simulink model "phdMain"  (R2023b)
settings: Solver=ode4  StartTime=0.0  StopTime=t.Data(end)  FixedStep=1e-3  RelTol=1e-3
values from neighbouring files (symbols this model uses):
  Am = T * Ac * inv(T)    [ref_model_mrac.m]
  Bm = T * Bc    [ref_model_mrac.m]
  Cm = eye(3)    [ref_model_mrac.m]
  Dm = zeros(3,1)    [ref_model_mrac.m]
undefined symbols (not defined in the file or in its folder): A_bar, AEFF, B_E, C_bar, C_T, Cd_neg, Cd_pos, DiscIntNeverNeededParam, Gamma, H, k, K, L_gain, L_STROKE, M, m3PsToLpm, P_return_Pa, P_supply_Pa, PA_Pa, PaToBar, PB_Pa, RHO, Ts, V01, V02, V_DEAD, v_mPs, W, xc_dot, xc_m
(part 1 of 3)
settings Model: PauseTimes=22  Creator=snr  LastModifiedBy=snr
settings DataIOCC: OutputOption=AdditionalOutputTimes  OutputTimes=1
settings OptimizationCC: BlockReduction=off  ConditionallyExecuteInputs=off
settings DebuggingCC: UnderSpecifiedDimensionMsg=warning

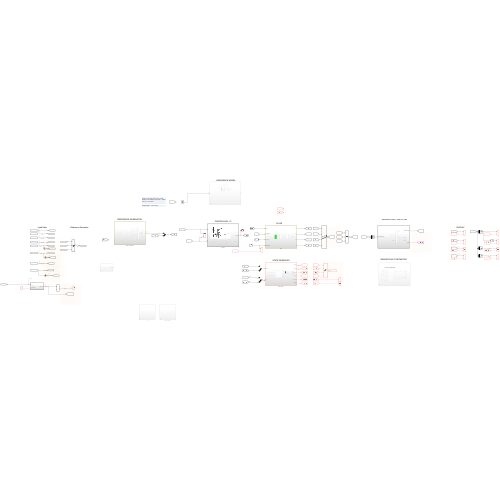
[thumbnail: Simulink's stored preview of the top-level diagram]
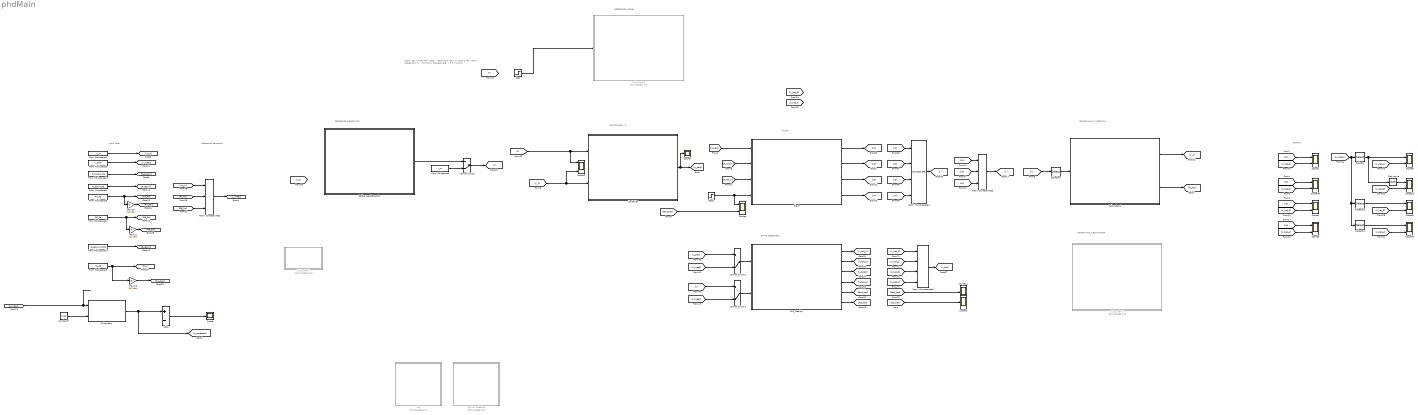
== system phdMain ==
  note: Kapalı Çevrim Faz Marjı (deg) > 6dB
      | Kapalı Çevrim Kazanç Marjı (dB) > 45deg
      | Aşım % < %5 olsun.
      |
      | Bantgenişliği > 5.5 Hz olsun
  note: Load Data
  note: PLANT
  note: CONTROLLER - PI
  note: DISPLAY
  note: Reference Generator
  note: SENSOR FAULT INJECTION
  note: STATE OBSERVER
  note: SENSOR FAULT ESTIMATOR
  note: REFERENCE GENERATOR
  note: REFERENCE MODEL
  Add5 : Sum  Inputs=+-
  Constant9 : Constant  Value=2.45
  Controller : Subsystem
  Derivative : Derivative
  EKF_Healthy : Subsystem
  From Workspace1 : FromWorkspace  VariableName=P_return_Pa
  From Workspace10 : FromWorkspace  VariableName=P_supply_Pa
  From Workspace11 : FromWorkspace  VariableName=PB_Pa
  From Workspace14 : FromWorkspace  VariableName=Q_return_m3Ps
  From Workspace2 : FromWorkspace  VariableName=r_m
  From Workspace3 : FromWorkspace  VariableName=u_perc
  From Workspace4 : FromWorkspace  VariableName=xc_m
  From Workspace5 : FromWorkspace  VariableName=PL_Pa
  From Workspace9 : FromWorkspace  VariableName=PA_Pa
  Gain19 : Gain  Gain=PaToBar
  Gain20 : Gain  Gain=PaToBar
  Gain21 : Gain  Gain=PaToBar
  Manual Switch : ManualSwitch  CurrentSetting=0
  Manual Switch1 : ManualSwitch  CurrentSetting=0
  Manual Switch2 : ManualSwitch  CurrentSetting=0
  Matrix Concatenate2 : Concatenate  NumInputs=3  Mode=Multidimensional array
  Matrix Concatenate3 : Concatenate  NumInputs=3  Mode=Multidimensional array
  Matrix Concatenate4 : Concatenate  NumInputs=4  Mode=Multidimensional array
  Matrix Concatenate5 : Concatenate  NumInputs=4  Mode=Multidimensional array
  Nguyen Observer : Subsystem  Commented=on
  Plant : Subsystem
  Reference_Generator : Subsystem
  Scope{,6..7,12} (4 alike) : Scope
  Scope{1..2,4..5,8..11,36} (9 alike) : Scope  NumInputPorts=2
  Scope3 : Scope  NumInputPorts=3
  Selector : Selector  InputPortWidth=3  IndexOptions=Index vector (dialog)  Indices=1  OutputSizes=1
  Selector1 : Selector  InputPortWidth=3  IndexOptions=Index vector (dialog)  Indices=3  OutputSizes=1
  Selector2 : Selector  InputPortWidth=3  IndexOptions=Index vector (dialog)  Indices=2  OutputSizes=1
  Selector4 : Selector  InputPortWidth=3  IndexOptions=Index vector (dialog)  Indices=1  OutputSizes=1
  Step : Step  After=10e-3  SampleTime=0
  Step2 : Step  Time=5  After=0  SampleTime=0
  Subsystem : Subsystem
  Subsystem1 : Subsystem
  Subsystem2 : Subsystem  Commented=on
  Subsystem3 : Subsystem  Commented=on
  Subsystem4 : Subsystem  Commented=on
  old : Subsystem  Commented=on
  wires:
  From Workspace3/1 -> [u_meas]  "u_real"
  From Workspace10/1 -> [P_supply]  "P_supply_Pa"
  From Workspace1/1 -> [P_return]  "P_return_Pa"
  From Workspace9/1 -> Gain20/1, [PA_Pa]  "PA_Pa"
  From Workspace11/1 -> Gain21/1, [PB_Pa]  "PB_Pa"
  From Workspace14/1 -> [Q_return]  "Q_return_m3Ps"
  From Workspace5/1 -> [P_L], Gain19/1  "P_L_Pa"
  Gain19/1 -> [P_L_bar]  "P_L_bar"
  Gain20/1 -> [PA_bar]  "PA_bar"
  Gain21/1 -> [PB_bar]  "PB_bar"
  [P_supply] -> Plant/2(P_supply_Pa)
  [P_return] -> Plant/3(P_return_Pa)
  Step2/1 -> Scope4/1, Plant/4(F_external_N)
  Plant/1(x1) -> [x1]
  Plant/2(x2) -> [x2]
  Plant/3(x3) -> [x3]
  Plant/4(x4) -> [x4]
  [x1] -> Matrix Concatenate3/1
  [x3] -> Matrix Concatenate3/2
  [x4] -> Matrix Concatenate3/3
  Matrix Concatenate3/1 -> [y]
  EKF_Healthy/1(x_hat_1) -> [x_hat_1]  "x_hat_1"
  EKF_Healthy/2(x_hat_2) -> [x_hat_2]  "x_hat_2"
  EKF_Healthy/3(x_hat_3) -> [x_hat_3]
  EKF_Healthy/4(x_hat_4) -> [x_hat_4]
  [x1] -> Matrix Concatenate4/1
  [x2] -> Matrix Concatenate4/2
  [x3] -> Matrix Concatenate4/3
  [x4] -> Matrix Concatenate4/4
  Matrix Concatenate4/1 -> [x]
  [x_hat_1] -> Matrix Concatenate5/1
  [x_hat_2] -> Matrix Concatenate5/2
  [x_hat_3] -> Matrix Concatenate5/3
  [x_hat_4] -> Matrix Concatenate5/4
  Matrix Concatenate5/1 -> [x_hat]
  EKF_Healthy/5(Fext_hat) -> [Fext_hat]
  EKF_Healthy/6(Qd_est) -> [Qd_hat]
  [x2] -> Scope36/1
  [x_hat_2] -> Scope36/2
  [y] -> Selector4/1
  Selector4/1 -> Subsystem1/1(Real_Cylinder_Pos)
  Subsystem1/1(Measured_Pos) -> [y_1]
  Subsystem1/2(fs_real) -> [fs_real]
  Controller/1(u_out_perc) -> Scope7/1, [u_perc]
  Step/1 -> Subsystem3/1(r)  "r"
  [y_1] -> Scope3/3, Controller/2(y)  "y_pid"
  Add5/1 -> Scope/1  "u_err"
  Subsystem/1(u_corrected) -> [u_corrected], Add5/1  "u_corrected"
  [u_meas] -> Subsystem/1(u)
  Constant9/1 -> Subsystem/2(u_perc_offset)
  [Fext_hat] -> Scope4/2
  Manual Switch/1 -> [r]  "r_m"
  Reference_Generator/1(r) -> Manual Switch/1  "r"
  From Workspace2/1 -> Manual Switch/2
  [x1] -> Scope1/1
  [x_hat_1] -> Scope1/2
  [x_hat_3] -> Scope2/2
  [x3] -> Scope2/1
  [x4] -> Scope5/1
  [x_hat_4] -> Scope5/2
  [Qd_hat] -> Scope6/1
  [PB_Pa] -> Matrix Concatenate2/3
  [PA_Pa] -> Matrix Concatenate2/2
  [xc_m] -> Matrix Concatenate2/1
  Matrix Concatenate2/1 -> [y_meas]
  Manual Switch1/1 -> EKF_Healthy/2(y_k)
  [y] -> Manual Switch1/1
  [y_meas] -> Manual Switch1/2
  Manual Switch2/1 -> EKF_Healthy/1(u_perc)
  [u_perc] -> Manual Switch2/1
  [u_meas] -> Manual Switch2/2
  [u_perc] -> Plant/1(u_perc)
  [r] -> Scope3/1, Controller/1(r)
  Selector1/1 -> Scope11/1  "P2_real"
  [x_hat_4] -> Scope11/2
  Selector/1 -> Derivative/1, Scope8/1
  [x_hat_1] -> Scope8/2
  [x_hat_2] -> Scope10/2
  Derivative/1 -> Scope10/1
  [x_hat_3] -> Scope9/2
  Selector2/1 -> Scope9/1  "P1_real"
  [y_meas] -> Selector1/1, Selector2/1, Selector/1
  From Workspace4/1 -> [xc_m]  "xc_m"
  [Fext_hat] -> Scope12/1

== system phdMain/Controller ==
  note: Kontrolcü kazançları Kp : 5 - Ki :40 test düzeneğinde, Sim ortamında uygunluk için böyle ayarladım
  note: Offset - Yapmaya İhtiyaç yok
  note: Integral Gain
  note: Proportional Gain
  r : Inport  OutDataTypeStr=double
  y : Inport  Port=2  OutDataTypeStr=double
  Add : Sum
  Add1 : Sum  Inputs=+-
  Add3 : Sum
  Constant : Constant  Value=10
  Constant1 : Constant  Value=5
  Constant2 : Constant  Value=0  OutDataTypeStr=double
  Gain1 : Gain  Gain=1000
  Integrator : Integrator
  Product : Product
  Product1 : Product
  Saturation : Saturate  UpperLimit=100  LowerLimit=-100
  u_out_perc : Outport  OutDataTypeStr=double
  wires:
  Constant/1 -> Product/1
  Constant1/1 -> Product1/1
  Add1/1 -> Product1/2, Product/2  "e"
  Product/1 -> Integrator/1
  Integrator/1 -> Add/2
  r/1 -> Add1/1  "r"
  Add/1 -> Gain1/1
  y/1 -> Add1/2
  Add3/1 -> Saturation/1
  Gain1/1 -> Add3/2
  Saturation/1 -> u_out_perc/1
  Product1/1 -> Add/1
  Constant2/1 -> Add3/1

== system phdMain/EKF_Healthy ==
  u_perc : Inport  OutDataTypeStr=double
  y_k : Inport  Port=2  OutDataTypeStr=double
  EKF_Discrete : MATLAB Function  TreatAsAtomicUnit=on  SystemSampleTime=1e-3
  Sel_d10 : Selector  InputPortWidth=6  IndexOptions=Index vector (dialog)  Indices=4  OutputSizes=1
  Sel_d7 : Selector  InputPortWidth=6  IndexOptions=Index vector (dialog)  Indices=1  OutputSizes=1
  Sel_d8 : Selector  InputPortWidth=6  IndexOptions=Index vector (dialog)  Indices=2  OutputSizes=1  RuntimeRangeChecks=on
  Sel_d9 : Selector  InputPortWidth=6  IndexOptions=Index vector (dialog)  Indices=3  OutputSizes=1
  Unit Delay : UnitDelay  SampleTime=1e-3  HasFrameUpgradeWarning=on
  x_hat_1 : Outport  OutDataTypeStr=double
  x_hat_2 : Outport  Port=2  OutDataTypeStr=double
  x_hat_3 : Outport  Port=3  OutDataTypeStr=double
  x_hat_4 : Outport  Port=4  OutDataTypeStr=double
  Fext_hat : Outport  Port=5  OutDataTypeStr=double
  Qd_est : Outport  Port=6  OutDataTypeStr=double
  wires:
  u_perc/1 -> EKF_Discrete/1(u_perc)  "u_perc"
  y_k/1 -> EKF_Discrete/2(y_k)
  EKF_Discrete/1(x_hat_out) -> Unit Delay/1
  Sel_d7/1 -> x_hat_1/1  "x_hat_1"
  Sel_d8/1 -> x_hat_2/1  "x_hat_2"
  Sel_d9/1 -> x_hat_3/1  "x_hat_3"
  Sel_d10/1 -> x_hat_4/1  "x_hat_4"
  EKF_Discrete/2(Fd_est) -> Fext_hat/1
  EKF_Discrete/3(Qd_est) -> Qd_est/1
  Unit Delay/1 -> Sel_d7/1, Sel_d10/1, Sel_d9/1, Sel_d8/1

== system phdMain/Nguyen Observer ==
  note: [1000; 1000; 1e-6; 1e-6]
  Add4 : Sum  Commented=on  Inputs=+-
  From Workspace13 : FromWorkspace  Commented=on  VariableName=P_return_Pa
  From Workspace16 : FromWorkspace  Commented=on  VariableName=P_supply_Pa
  From Workspace17 : FromWorkspace  Commented=on  VariableName=PB_Pa
  From Workspace18 : FromWorkspace  Commented=on  VariableName=PA_Pa
  From14 : From  Commented=on  GotoTag=u_perc
  From15 : From  Commented=on  GotoTag=xc_sim
  From20 : From  Commented=on  GotoTag=xc_dot_sim
  From29 : From  Commented=on  GotoTag=x1_hat
  From32 : From  Commented=on  GotoTag=xc_sim
  From33 : From  Commented=on  GotoTag=x2_hat
  From36 : From  Commented=on  GotoTag=fs_hat
  From37 : From  Commented=on  GotoTag=PA_sim_Pa
  From38 : From  Commented=on  GotoTag=x3_hat
  From40 : From  Commented=on  GotoTag=xc_dot_sim
  Gain15 : Gain  Commented=on  Gain=[1000; 1000; 1e-6; 1e-6]
  Goto21 : Goto  Commented=on  GotoTag=x1_hat
  Goto22 : Goto  Commented=on  GotoTag=x3_hat
  Goto26 : Goto  Commented=on  GotoTag=fs_hat
  Goto27 : Goto  Commented=on  GotoTag=x4_hat
  Goto28 : Goto  Commented=on  GotoTag=x2_hat
  Matrix Concatenate : Concatenate  Commented=on  NumInputs=4  Mode=Multidimensional array
  Nguyen_Observer : Subsystem  Commented=on
  Scope12 : Scope  Commented=on  NumInputPorts=2
  Scope17 : Scope  Commented=on  NumInputPorts=2
  Scope18 : Scope  Commented=on
  Scope19 : Scope  Commented=on
  Scope20 : Scope  Commented=on  NumInputPorts=2
  Selector : Selector  Commented=on  InputPortWidth=5  IndexOptions=Index vector (dialog)  Indices=1  OutputSizes=1
  Selector1 : Selector  Commented=on  InputPortWidth=5  IndexOptions=Index vector (dialog)  Indices=2  OutputSizes=1
  Selector2 : Selector  Commented=on  InputPortWidth=5  IndexOptions=Index vector (dialog)  Indices=3  OutputSizes=1
  Selector3 : Selector  Commented=on  InputPortWidth=5  IndexOptions=Index vector (dialog)  Indices=4  OutputSizes=1
  Selector4 : Selector  Commented=on  InputPortWidth=5  IndexOptions=Index vector (dialog)  Indices=5  OutputSizes=1
  Zero-Order Hold3 : ZeroOrderHold  Commented=on  SampleTime=Ts
  wires:
  From Workspace13/1 -> Nguyen_Observer/3(P_return)
  Add4/1 -> Scope19/1
  From Workspace17/1 -> Matrix Concatenate/4
  Selector4/1 -> Goto26/1
  From14/1 -> Nguyen_Observer/1(u_perc)  "u_perc"
  Selector2/1 -> Goto22/1
  Matrix Concatenate/1 -> Zero-Order Hold3/1
  From38/1 -> Scope20/2
  From Workspace16/1 -> Nguyen_Observer/2(P_supply)
  From32/1 -> Add4/1, Scope12/1
  Zero-Order Hold3/1 -> Gain15/1
  From36/1 -> Scope18/1
  From40/1 -> Scope17/1
  Gain15/1 -> Nguyen_Observer/4(y)
  From20/1 -> Matrix Concatenate/2
  From15/1 -> Matrix Concatenate/1
  Selector/1 -> Goto21/1
  Selector3/1 -> Goto27/1
  From37/1 -> Scope20/1  "PA_sim_Pa"
  Selector1/1 -> Goto28/1
  From Workspace18/1 -> Matrix Concatenate/3
  Nguyen_Observer/1(xbar_hat_safe) -> Selector4/1, Selector3/1, Selector2/1, Selector1/1, Selector/1
  From33/1 -> Scope17/2
  From29/1 -> Add4/2, Scope12/2

== system phdMain/Plant ==
  u_perc : Inport  OutDataTypeStr=double
  P_supply_Pa : Inport  Port=2
  P_return_Pa : Inport  Port=3
  F_external_N : Inport  Port=4
  Cylinder_Dynamics : Subsystem
  Pressure_Dynamics : Subsystem
  Subsystem1 : Subsystem
  x1 : Outport
  x2 : Outport  Port=2
  x3 : Outport  Port=3
  x4 : Outport  Port=4
  wires:
  Cylinder_Dynamics/1(xc_sim) -> [xc_sim]  "xc_sim_m"
  [xc_sim] -> Pressure_Dynamics/3(xc)
  P_supply_Pa/1 -> Subsystem1/2(P_supply)
  [PA_sim_Pa] -> Subsystem1/4(PA_sim_Pa)  "PA_sim_Pa"
  [PB_sim_Pa] -> Subsystem1/5(PB_sim_Pa)  "PB_sim_Pa"
  [PB_sim_Pa] -> Cylinder_Dynamics/2(PB_sim_Pa)  "PB_sim_Pa"
  Pressure_Dynamics/1(PA_sim) -> [PA_sim_Pa]  "PA_sim_Pa"
  Cylinder_Dynamics/3(xc_ddot_sim) -> [xc_ddot_sim]  "xc_ddot_sim_mPs2"
  Cylinder_Dynamics/2(xc_dot_sim) -> [xc_dot_sim]  "xc_dot_sim_mPs"
  [xc_dot_sim] -> Pressure_Dynamics/2(xc_dot)
  [PA_sim_Pa] -> Cylinder_Dynamics/1(PA_sim_Pa)  "PA_sim_Pa"
  Pressure_Dynamics/2(PB_sim) -> [PB_sim_Pa]  "PB_sim_Pa"
  Subsystem1/1(q_withLeaks) -> [Q_Bus]
  [Q_Bus] -> Pressure_Dynamics/1(q)
  u_perc/1 -> Subsystem1/1(u_perc)  "u_perc"
  P_return_Pa/1 -> Subsystem1/3(P_return)
  F_external_N/1 -> Cylinder_Dynamics/3(F_ext)
  [xc_sim] -> x1/1  "xc_sim"
  [xc_dot_sim] -> x2/1  "xc_dot_sim"
  [PA_sim_Pa] -> x3/1  "PA_sim_Pa"
  [PB_sim_Pa] -> x4/1  "PB_sim_Pa"

== system phdMain/Reference_Generator ==
  Constant : Constant  OutDataTypeStr=uint8
  Constant1 : Constant  Commented=on  Value=30  OutDataTypeStr=double
  Constant2 : Constant  Commented=on  OutDataTypeStr=double
  Constant3 : Constant  Commented=on  Value=0  OutDataTypeStr=double
  Constant4 : Constant  Value=0
  From Workspace14 : FromWorkspace  VariableName=r_m
  Gain : Gain
  Multiport Switch : MultiPortSwitch  DataPortOrder=Zero-based contiguous  DataPortForDefault=Additional data port  DiagnosticForDefault=None  zeroidx=on  OutDataTypeStr=double  SaturateOnIntegerOverflow=off  InputSameDT=off
  Pulse Generator : DiscretePulseGenerator  PulseType=Time based  Amplitude=20e-3  Period=4  PulseWidth=25
  Scope : Scope
  Sine Wave : Sin  Amplitude=30e-3  Frequency=pi*0.5  SampleTime=0
  Sine_Generator : Subsystem  Commented=on
  r : Outport  OutDataTypeStr=double
  wires:
  From Workspace14/1 -> Multiport Switch/2  "r_m"
  Constant/1 -> Multiport Switch/1
  Constant1/1 -> Sine_Generator/1(Amp_mm)
  Constant2/1 -> Sine_Generator/2(f_Hz)
  Constant3/1 -> Sine_Generator/3(phi_deg)
  Pulse Generator/1 -> Gain/1
  Multiport Switch/1 -> Scope/1, r/1
  Constant4/1 -> Multiport Switch/5
  Sine Wave/1 -> Multiport Switch/3
  Gain/1 -> Multiport Switch/4

== system phdMain/Subsystem ==
  u : Inport  OutDataTypeStr=double
  u_perc_offset : Inport  Port=2  OutDataTypeStr=double
  Add : Sum  Inputs=+-
  u_corrected : Outport
  wires:
  u/1 -> Add/1
  u_perc_offset/1 -> Add/2
  Add/1 -> u_corrected/1

== system phdMain/Subsystem1 ==
  Real_Cylinder_Pos : Inport  OutDataTypeStr=double
  Add4 : Sum
  Fault_Injection : Subsystem  Commented=on
  Measured_Pos : Outport  OutDataTypeStr=double
  fs_real : Outport  Port=2  OutDataTypeStr=double
  wires:
  Fault_Injection/1(fs) -> [fs_real], Add4/1
  Real_Cylinder_Pos/1 -> Add4/2
  Add4/1 -> Measured_Pos/1  "y_1"
  [fs_real] -> fs_real/1

== system phdMain/Subsystem2 ==
  note: FAULT ESTIMATOR
  From14 : From  Commented=on  GotoTag=u_perc
  From15 : From  Commented=on  GotoTag=PA_sim_Pa
  From20 : From  Commented=on  GotoTag=PB_sim_Pa
  From29 : From  Commented=on  GotoTag=fs_real
  From33 : From  Commented=on  GotoTag=xc_dot_sim
  Scope12 : Scope  Commented=on  NumInputPorts=3
  Scope17 : Scope  Commented=on  NumInputPorts=3
  Subsystem3 : Subsystem  Commented=on
  wires:
  Subsystem3/2(Out1) -> Scope17/1
  From20/1 -> Subsystem3/3(PB_Pa)  "PB_sim_Pa"
  From29/1 -> Subsystem3/5(fs_real)
  From14/1 -> Subsystem3/1(u_real)  "u_perc"
  From33/1 -> Scope17/2
  From15/1 -> Subsystem3/2(PA_Pa)
  Subsystem3/1(x_bar) -> Scope12/2  "x_bar"

== system phdMain/Subsystem3 ==
  r : Inport  OutDataTypeStr=double
  Add : Sum  Inputs=+-
  Gain : Gain
  Scope10 : Scope  NumInputPorts=2
  Scope11 : Scope
  Scope12 : Scope
  Scope13 : Scope
  Scope8 : Scope  NumInputPorts=2
  Scope9 : Scope  NumInputPorts=2
  Selector : Selector  InputPortWidth=3  IndexOptions=Index vector (dialog)  Indices=1  OutputSizes=1
  Selector1 : Selector  InputPortWidth=3  IndexOptions=Index vector (dialog)  Indices=2  OutputSizes=1
  Selector2 : Selector  InputPortWidth=3  IndexOptions=Index vector (dialog)  Indices=3  OutputSizes=1
  State-Space : StateSpace  A=Am  B=Bm  C=Cm  D=Dm  InitialCondition=[0;0;0]
  Out1 : Outport
  wires:
  r/1 -> State-Space/1, Scope12/1, Scope8/1  "r"
  Selector1/1 -> Scope13/1, Scope9/1
  [x2] -> Scope9/2
  Gain/1 -> Scope10/1
  State-Space/1 -> Selector2/1, Selector1/1, Selector/1
  Selector/1 -> Scope8/2  "y_m"
  Selector2/1 -> Scope11/1, Gain/1
  Add/1 -> Scope10/2

== system phdMain/Subsystem4 ==
  In1 : Inport
  Add : Sum
  Constant : Constant
  Constant1 : Constant  Value=100
  Relational Operator : RelationalOperator  OutDataTypeStr=boolean  RndMeth=Simplest  InputSameDT=off
  Saturation : Saturate  UpperLimit=100  LowerLimit=0
  Switch : Switch  Criteria=u2 ~= 0  SaturateOnIntegerOverflow=off  InputSameDT=off
  Unit Delay : UnitDelay  SampleTime=-1  HasFrameUpgradeWarning=on
  u_perc_offset : Outport
  wires:
  Constant/1 -> Add/1
  Add/1 -> Unit Delay/1, Saturation/1
  Unit Delay/1 -> Add/2
  Saturation/1 -> Relational Operator/1
  Constant1/1 -> Relational Operator/2
  Relational Operator/1 -> Switch/2
  In1/1 -> Switch/1

== system phdMain/old ==
  Bus Creator1 : BusCreator  Commented=on  Inputs=3
  Constant10 : Constant  Commented=on  Value=mean(P_supply_Pa)
  Constant4 : Constant  Commented=on  Value=mean(P_return_Pa)
  Constant6 : Constant  Commented=on  Value=mean(P_supply_Pa)
  Constant9 : Constant  Commented=on  Value=mean(P_return_Pa)
  Flow_Calc_NoLeak : Subsystem  Commented=on
  Flow_Calc_WithLeak : Subsystem  Commented=on
  From Workspace13 : FromWorkspace  Commented=on  VariableName=P_supply_Pa
  From Workspace8 : FromWorkspace  Commented=on  VariableName=P_return_Pa
  From13 : From  Commented=on  GotoTag=PA_sim_Pa
  From14 : From  Commented=on  GotoTag=PB_sim_Pa
  From15 : From  Commented=on  GotoTag=u_perc
  From23 : From  Commented=on  GotoTag=PA_sim_Pa
  From26 : From  Commented=on  GotoTag=PB_sim_Pa
  From29 : From  Commented=on  GotoTag=Q_return
  From32 : From  Commented=on  GotoTag=q_withLeaks
  From37 : From  Commented=on  GotoTag=xv
  From38 : From  Commented=on  GotoTag=PA_sim_Pa
  From39 : From  Commented=on  GotoTag=PB_sim_Pa
  From40 : From  Commented=on  GotoTag=xv
  From43 : From  Commented=on  GotoTag=xv
  Gain15 : Gain  Commented=on  Gain=50E-3/100
  Gain16 : Gain  Commented=on  Gain=m3PsToLpm
  Gain17 : Gain  Commented=on  Gain=m3PsToLpm
  Goto21 : Goto  Commented=on  GotoTag=xv
  Goto26 : Goto  Commented=on  GotoTag=q_withLeaks
  Goto27 : Goto  Commented=on  GotoTag=q_NoLeaks
  MATLAB Function2 : MATLAB Function  Commented=on  TreatAsAtomicUnit=on
  Scope14 : Scope  NumInputPorts=2
  Scope17 : Scope  Commented=on  NumInputPorts=2
  ServoValve_Dynamics : Subsystem  Commented=on
  wires:
  Constant9/1 -> MATLAB Function2/3(P_T)
  From32/1 -> Scope14/2
  Constant4/1 -> Flow_Calc_WithLeak/3(P_return)
  From26/1 -> MATLAB Function2/5(P_B)  "PB_sim_Pa"
  From Workspace13/1 -> Flow_Calc_NoLeak/2(P_supply)
  From29/1 -> Gain17/1
  Gain15/1 -> MATLAB Function2/1(xv)
  Bus Creator1/1 -> Scope14/1
  From37/1 -> Flow_Calc_WithLeak/1(xv)
  Constant10/1 -> MATLAB Function2/2(P_P)
  From Workspace8/1 -> Flow_Calc_NoLeak/3(P_return)
  MATLAB Function2/3(Q_RETURN) -> Gain16/1, Bus Creator1/3  "Q_RETURN_lpm"
  From23/1 -> MATLAB Function2/4(P_A)  "PA_sim_Pa"
  Gain16/1 -> Scope17/2  "Q_RETURN_lpm"
  MATLAB Function2/1(Q1) -> Bus Creator1/1  "q1"
  MATLAB Function2/2(Q2) -> Bus Creator1/2  "q2"
  From14/1 -> Flow_Calc_WithLeak/5(P_2)  "P_2_sim"
  From39/1 -> Flow_Calc_NoLeak/5(P_2)  "P_2_sim"
  Flow_Calc_NoLeak/1(Q) -> Goto27/1
  Flow_Calc_WithLeak/1(q_withLeaks) -> Goto26/1
  From40/1 -> Flow_Calc_NoLeak/1(xv)
  [u_sim] -> Gain15/1
  Constant6/1 -> Flow_Calc_WithLeak/2(P_supply)
  From38/1 -> Flow_Calc_NoLeak/4(P_1)  "P_1_sim"
  From13/1 -> Flow_Calc_WithLeak/4(P_1)  "P_1_sim"
  Gain17/1 -> Scope17/1  "Q_RETURN_lpmREAL"
  ServoValve_Dynamics/1(xv) -> Goto21/1  "xv"
  From15/1 -> ServoValve_Dynamics/1(u)  "u_sim"

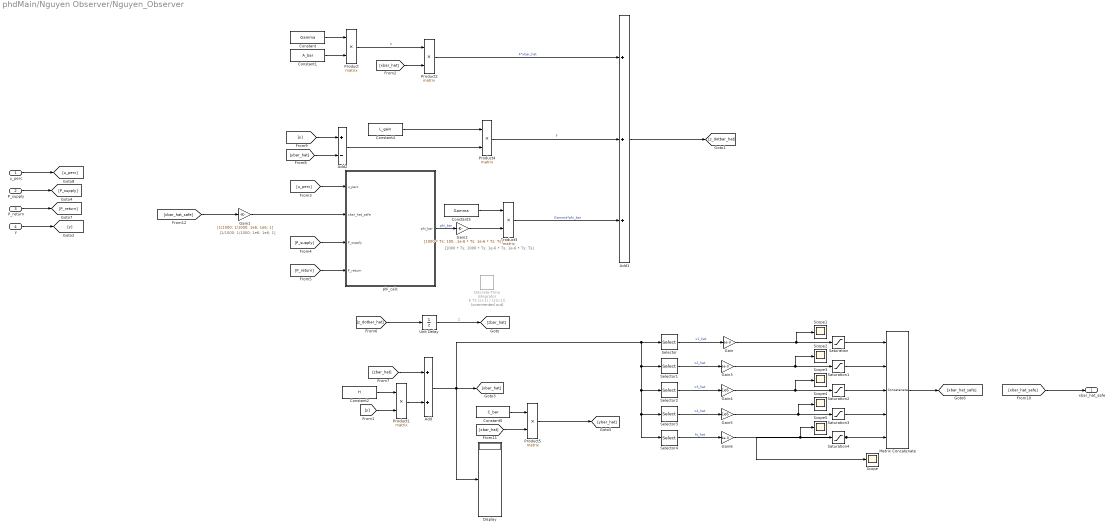
== system phdMain/Nguyen Observer/Nguyen_Observer ==
  note: [1000 * Ts; 1000 * Ts; 1e-6 * Ts; 1e-6 * Ts; Ts]
  note: [1/1000; 1/1000; 1e6; 1e6; 1]
  u_perc : Inport  PortDimensions=[1,1]
  P_supply : Inport  Port=2  OutDataTypeStr=double
  P_return : Inport  Port=3  OutDataTypeStr=double
  y : Inport  Port=4  PortDimensions=[4,1]
  Add : Sum
  Add1 : Sum  Inputs=+++
  Add2 : Sum  Inputs=+-
  Constant : Constant  Value=Gamma
  Constant1 : Constant  Value=A_bar
  Constant2 : Constant  Value=H
  Constant3 : Constant  Value=Gamma
  Constant4 : Constant  Value=L_gain
  Constant5 : Constant  Value=C_bar
  Discrete-Time Integrator : DiscreteIntegrator  Commented=on  IntegratorMethod=Integration: Trapezoidal  InitialCondition=[0,0,PA_Pa.Data(1)*1e-6,PB_Pa.Data(1)*1e-6,0]'  SampleTime=-1  ICPrevOutput=DiscIntNeverNeededParam  ICPrevScaledInput=DiscIntNeverNeededParam
  Display : Display
  Gain : Gain  Gain=1e-3
  Gain1 : Gain  Gain=[1/1000; 1/1000; 1e6; 1e6; 1]
  Gain2 : Gain  Gain=[1000 * Ts; 1000 * Ts; 1e-6 * Ts; 1e-6 * Ts; Ts]
  Gain3 : Gain  Gain=1e-3
  Gain4 : Gain  Gain=1e6
  Gain5 : Gain  Gain=1e6
  Gain6 : Gain  Gain=1e-3
  Matrix Concatenate : Concatenate  NumInputs=5  Mode=Multidimensional array
  Product{,1..5} (6 alike) : Product  Multiplication=Matrix(*)
  Saturation : Saturate  UpperLimit=L_STROKE  LowerLimit=-L_STROKE
  Saturation1 : Saturate  UpperLimit=2  LowerLimit=-2
  Saturation2 : Saturate  UpperLimit=200e5  LowerLimit=4e5
  Saturation3 : Saturate  UpperLimit=200e5  LowerLimit=4e5
  Saturation4 : Saturate  UpperLimit=L_STROKE  LowerLimit=-L_STROKE
  Scope{,1..5} (6 alike) : Scope
  Selector : Selector  InputPortWidth=5  IndexOptions=Index vector (dialog)  Indices=1  OutputSizes=1
  Selector1 : Selector  InputPortWidth=5  IndexOptions=Index vector (dialog)  Indices=2  OutputSizes=1
  Selector2 : Selector  InputPortWidth=5  IndexOptions=Index vector (dialog)  Indices=3  OutputSizes=1
  Selector3 : Selector  InputPortWidth=5  IndexOptions=Index vector (dialog)  Indices=4  OutputSizes=1
  Selector4 : Selector  InputPortWidth=5  IndexOptions=Index vector (dialog)  Indices=5  OutputSizes=1
  Unit Delay : UnitDelay  InitialCondition=[0,0,PA_Pa.Data(1)*1e-6,PB_Pa.Data(1)*1e-6,0]'  SampleTime=Ts  HasFrameUpgradeWarning=on
  phi_calc : Subsystem
  xbar_hat_safe : Outport
  wires:
  [y] -> Add2/1
  Product3/1 -> Add1/3  "Gamma*phi_bar"
  [u_perc] -> phi_calc/1(u_perc)
  Add2/1 -> Product4/2
  u_perc/1 -> [u_perc]
  Constant3/1 -> Product3/1
  Unit Delay/1 -> [zbar_hat]  "z"
  [ybar_hat] -> Add2/2
  Constant2/1 -> Product1/1
  Product/1 -> Product2/1  "F"
  [P_return] -> phi_calc/4(P_return)
  Constant1/1 -> Product/2
  Product2/1 -> Add1/1  "F*xbar_hat"
  Constant/1 -> Product/1
  [xbar_hat] -> Product2/2
  P_return/1 -> [P_return]
  [y] -> Product1/2
  [zbar_hat] -> Add/1
  y/1 -> [y]
  Add1/1 -> [z_dotbar_hat]
  Product4/1 -> Add1/2  "F"
  Product1/1 -> Add/2
  P_supply/1 -> [P_supply]
  phi_calc/1(phi_bar) -> Gain2/1  "phi_bar"
  [P_supply] -> phi_calc/3(P_supply)
  [z_dotbar_hat] -> Unit Delay/1
  [xbar_hat_safe] -> xbar_hat_safe/1
  Constant5/1 -> Product5/1
  [xbar_hat] -> Product5/2
  Product5/1 -> [ybar_hat]
  Selector3/1 -> Gain5/1  "x4_hat"
  Selector2/1 -> Gain4/1  "x3_hat"
  Selector1/1 -> Gain3/1  "x2_hat"
  Saturation/1 -> Matrix Concatenate/1
  Saturation1/1 -> Matrix Concatenate/2
  Saturation2/1 -> Matrix Concatenate/3
  Saturation3/1 -> Matrix Concatenate/4
  Saturation4/1 -> Scope/1, Matrix Concatenate/5
  Matrix Concatenate/1 -> [xbar_hat_safe]
  Selector4/1 -> Gain6/1  "fs_hat"
  Selector/1 -> Gain/1  "x1_hat"
  Constant4/1 -> Product4/1
  Add/1 -> Selector3/1, Selector4/1, Selector2/1, Selector1/1, Selector/1, [xbar_hat], Display/1
  [xbar_hat_safe] -> Gain1/1
  Gain1/1 -> phi_calc/2(xbar_hat_safe)
  Gain2/1 -> Product3/2
  Gain/1 -> Scope1/1, Saturation/1
  Gain3/1 -> Scope2/1, Saturation1/1
  Gain4/1 -> Saturation2/1, Scope3/1
  Gain5/1 -> Saturation3/1, Scope4/1
  Gain6/1 -> Scope5/1, Saturation4/1

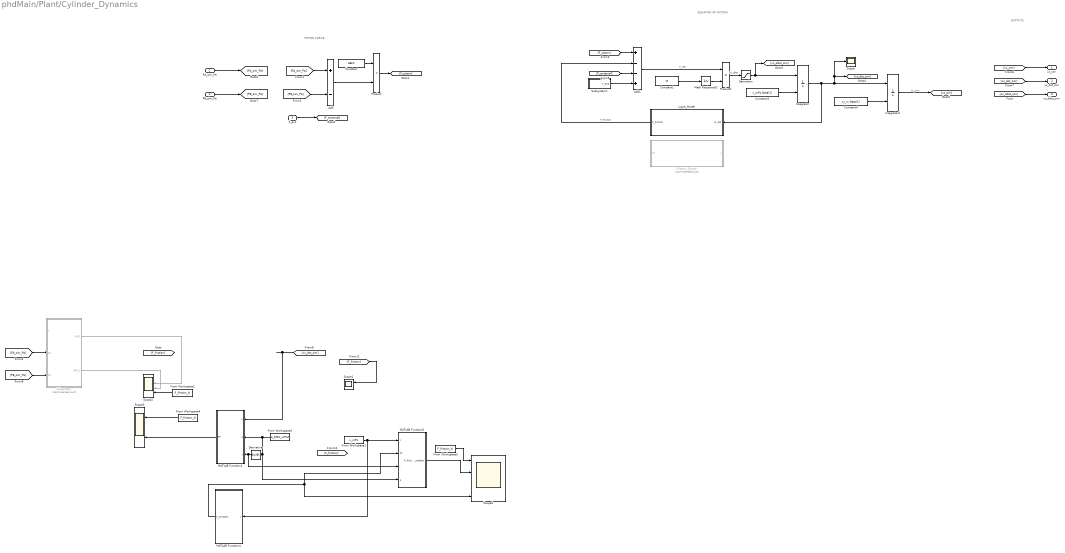
== system phdMain/Plant/Cylinder_Dynamics ==
  note: PISTON FORCE
  note: EQUATION OF MOTION
  note: OUTPUTS
  PA_sim_Pa : Inport  OutDataTypeStr=double
  PB_sim_Pa : Inport  Port=2  OutDataTypeStr=double
  F_ext : Inport  Port=3  OutDataTypeStr=double
  Add : Sum  Inputs=+-
  Add1 : Sum  Inputs=+--+
  Constant : Constant  Value=AEFF  OutDataTypeStr=double
  Constant1 : Constant  Value=M  OutDataTypeStr=double
  Constant3 : Constant  Value=v_mPs.Data(1)
  Constant4 : Constant  Value=xc_m.Data(1)
  Derivative : Derivative
  Friction_Simple : MATLAB Function  Commented=on  TreatAsAtomicUnit=on
  From Workspace1 : FromWorkspace  VariableName=v_mPs
  From Workspace2 : FromWorkspace  VariableName=F_friction_N
  From Workspace3 : FromWorkspace  VariableName=F_friction_N
  From Workspace4 : FromWorkspace  VariableName=F_friction_N
  From Workspace5 : FromWorkspace  VariableName=a_RMC_mPs2
  Integrator : Integrator  InitialConditionSource=external  InitialCondition=xc_dot(1)  UpperSaturationLimit=4  LowerSaturationLimit=-4
  Integrator2 : Integrator  InitialConditionSource=external  InitialCondition=xc_dot(1)  LimitOutput=on  UpperSaturationLimit=0.09580  LowerSaturationLimit=-0.09580
  Lugre_Model : Subsystem
  MATLAB Function1 : MATLAB Function  TreatAsAtomicUnit=on
  MATLAB Function3 : MATLAB Function  TreatAsAtomicUnit=on
  MATLAB Function4 : MATLAB Function  TreatAsAtomicUnit=on
  Math Reciprocal2 : Math  Operator=reciprocal  SignedPower=on
  Product : Product
  Product1 : Product
  Saturation : Saturate  UpperLimit=100  LowerLimit=-100
  Scope : Scope
  Scope1 : Scope  NumInputPorts=2
  Scope2 : Scope  NumInputPorts=6
  Scope3 : Scope  NumInputPorts=2
  Scope4 : Scope  NumInputPorts=4
  Subsystem : Subsystem  Commented=on
  Subsystem1 : Subsystem
  xc_sim : Outport  OutDataTypeStr=double
  xc_dot_sim : Outport  Port=2  OutDataTypeStr=double
  xc_ddot_sim : Outport  Port=3  OutDataTypeStr=double
  wires:
  [PB_sim_Pa] -> Add/2
  [PA_sim_Pa] -> Add/1
  Add/1 -> Product/2
  Constant/1 -> Product/1
  Math Reciprocal2/1 -> Product1/2
  Product1/1 -> Saturation/1  "xc_ddot"
  Product/1 -> [F_piston]
  F_ext/1 -> [F_external]
  Add1/1 -> Product1/1  "F_net"
  Constant3/1 -> Integrator/2
  Integrator/1 -> Integrator2/1, Scope/1, [xc_dot_sim], Lugre_Model/1(xc_dot)
  Constant4/1 -> Integrator2/2
  Integrator2/1 -> [xc_sim]  "xc_sim"
  [xc_sim] -> xc_sim/1
  [xc_dot_sim] -> xc_dot_sim/1
  [xc_dot_sim] -> MATLAB Function1/1(v)
  [xc_ddot_sim] -> xc_ddot_sim/1
  Saturation/1 -> [xc_ddot_sim], Integrator/1
  [F_external] -> Add1/3
  [F_piston] -> Add1/1
  ? -> Scope2/1, [F_friction]  "F_friction"
  From Workspace2/1 -> Scope2/5
  Subsystem1/1(F_end) -> Add1/4
  PA_sim_Pa/1 -> [PA_sim_Pa]
  PB_sim_Pa/1 -> [PB_sim_Pa]
  [PA_sim_Pa] -> Subsystem/2(pa)
  [PB_sim_Pa] -> Subsystem/3(pb)
  Constant1/1 -> Math Reciprocal2/1
  Subsystem/2(FRIC1) -> Scope2/4
  Subsystem/1(FRIC) -> Scope2/3
  Derivative/1 -> MATLAB Function3/3(j), MATLAB Function1/3(j)
  From Workspace4/1 -> Scope3/1
  MATLAB Function1/1(FF) -> Scope3/2
  From Workspace5/1 -> MATLAB Function3/4(a), Derivative/1, MATLAB Function1/2(a)
  [F_friction] -> Scope1/1
  From Workspace1/1 -> MATLAB Function4/1(v), MATLAB Function3/1(v)
  MATLAB Function3/1(F_friction_nodelay) -> Scope4/2
  From Workspace3/1 -> Scope4/1
  MATLAB Function4/1(F_stribeck) -> MATLAB Function3/2(FF), Scope4/4
  Lugre_Model/1(F_friction) -> Add1/2  "F_friction"

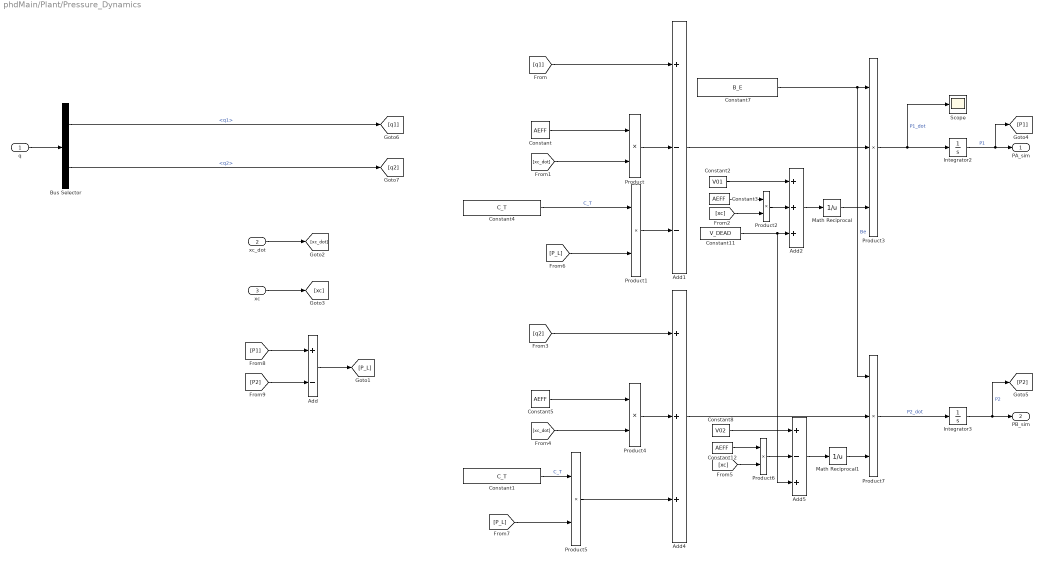
== system phdMain/Plant/Pressure_Dynamics ==
  q : Inport  OutDataTypeStr=double
  xc_dot : Inport  Port=2  OutDataTypeStr=double
  xc : Inport  Port=3  OutDataTypeStr=double
  Add : Sum  Inputs=+-
  Add1 : Sum  Inputs=+--
  Add2 : Sum  Inputs=+++
  Add4 : Sum  Inputs=+++
  Add5 : Sum  Inputs=+-+
  Bus Selector : BusSelector  OutputSignals=q1,q2
  Constant{,3,5,12} (4 alike) : Constant  Value=AEFF  OutDataTypeStr=double
  Constant1 : Constant  Value=C_T  OutDataTypeStr=double
  Constant11 : Constant  Value=V_DEAD  OutDataTypeStr=double
  Constant2 : Constant  Value=V01  OutDataTypeStr=double
  Constant4 : Constant  Value=C_T  OutDataTypeStr=double
  Constant7 : Constant  Value=B_E  OutDataTypeStr=double
  Constant8 : Constant  Value=V02  OutDataTypeStr=double
  Integrator2 : Integrator  InitialCondition=PA_Pa.Data(1)  LimitOutput=on  UpperSaturationLimit=200e5  LowerSaturationLimit=4e5
  Integrator3 : Integrator  InitialCondition=PB_Pa.Data(1)  LimitOutput=on  UpperSaturationLimit=200e5  LowerSaturationLimit=4e5
  Math Reciprocal : Math  Operator=reciprocal  SignedPower=on
  Math Reciprocal1 : Math  Operator=reciprocal  SignedPower=on
  Product{,1..2,4..6} (6 alike) : Product
  Product3 : Product  Inputs=3
  Product7 : Product  Inputs=3
  Scope : Scope
  PA_sim : Outport  OutDataTypeStr=double
  PB_sim : Outport  Port=2  OutDataTypeStr=double
  wires:
  q/1 -> Bus Selector/1
  xc_dot/1 -> [xc_dot]
  [xc_dot] -> Product/2
  Constant/1 -> Product/1
  Integrator2/1 -> [P1], PA_sim/1  "P1"
  [P_L] -> Product1/2
  Product/1 -> Add1/2
  [q1] -> Add1/1
  xc/1 -> [xc]
  Constant2/1 -> Add2/1
  Product2/1 -> Add2/2
  [xc] -> Product2/2
  Constant3/1 -> Product2/1
  Add2/1 -> Math Reciprocal/1
  Product3/1 -> Integrator2/1, Scope/1  "P1_dot"
  Math Reciprocal/1 -> Product3/3
  Add1/1 -> Product3/2
  Constant7/1 -> Product7/1, Product3/1  "Be"
  Constant4/1 -> Product1/1  "C_T"
  [xc_dot] -> Product4/2
  Product4/1 -> Add4/2
  Add4/1 -> Product7/2
  Integrator3/1 -> [P2], PB_sim/1  "P2"
  [P_L] -> Product5/2
  Constant5/1 -> Product4/1
  Add5/1 -> Math Reciprocal1/1
  [q2] -> Add4/1
  Math Reciprocal1/1 -> Product7/3
  Product7/1 -> Integrator3/1  "P2_dot"
  [xc] -> Product6/2
  Constant8/1 -> Add5/1
  Constant12/1 -> Product6/1
  Product6/1 -> Add5/2
  Bus Selector/2 -> [q2]  "<q2>"
  Bus Selector/1 -> [q1]  "<q1>"
  [P2] -> Add/2
  [P1] -> Add/1
  Add/1 -> [P_L]
  Constant1/1 -> Product5/1  "C_T"
  Product5/1 -> Add4/3
  Product1/1 -> Add1/3
  Constant11/1 -> Add5/3, Add2/3

== system phdMain/Plant/Subsystem1 ==
  u_perc : Inport  OutDataTypeStr=double
  P_supply : Inport  Port=2  OutDataTypeStr=double
  P_return : Inport  Port=3  OutDataTypeStr=double
  PA_sim_Pa : Inport  Port=4  OutDataTypeStr=double
  PB_sim_Pa : Inport  Port=5  OutDataTypeStr=double
  Bus Creator4 : BusCreator  Inputs=2
  Constant1 : Constant  Value=0.01
  Constant2 : Constant  Value=25e-3
  Constant4 : Constant  Value=k
  Constant7 : Constant  Value=K
  Dead Zone : DeadZone  LowerValue=-0.02  UpperValue=0.02
  Dead Zone1 : DeadZone  LowerValue=-0.02  UpperValue=0.02
  From Workspace2 : FromWorkspace  VariableName=Q_return_m3Ps
  Gain1 : Gain  Gain=m3PsToLpm
  Gain2 : Gain  Gain=m3PsToLpm
  MATLAB Function : MATLAB Function  TreatAsAtomicUnit=on
  Product : Product  Inputs=3
  Scope1 : Scope  NumInputPorts=2
  Terminator : Terminator
  Valve Dynamics : TransferFcn  Numerator=[2.0884e+06]  Denominator=[1 2*1*1.4451e+03 2.0884e+06]
  q_withLeaks : Outport  OutDataTypeStr=double
  wires:
  PA_sim_Pa/1 -> [P_A]
  P_supply/1 -> [P_supply]
  P_return/1 -> [P_return]
  PB_sim_Pa/1 -> [P_B]
  u_perc/1 -> [u_perc]
  [P_supply] -> MATLAB Function/2(Ps)
  [P_return] -> MATLAB Function/3(Pr)
  [P_A] -> MATLAB Function/4(P1)
  [P_B] -> MATLAB Function/5(P2)
  Bus Creator4/1 -> q_withLeaks/1
  MATLAB Function/1(Q1) -> Bus Creator4/1  "q1"
  MATLAB Function/2(Q2) -> Bus Creator4/2  "q2"
  Constant2/1 -> Product/1
  Product/1 -> MATLAB Function/1(x)  "i"
  Constant1/1 -> Product/2
  Constant4/1 -> MATLAB Function/7(k)
  Constant7/1 -> MATLAB Function/6(K)
  [u_perc] -> Dead Zone1/1
  From Workspace2/1 -> Gain1/1
  Gain2/1 -> Scope1/1  "Q_return_calc_lpm"
  Gain1/1 -> Scope1/2  "Q_return_lpm"
  MATLAB Function/3(QR) -> Terminator/1
  Dead Zone/1 -> Valve Dynamics/1
  Dead Zone1/1 -> Product/3

== system phdMain/Reference_Generator/Sine_Generator ==
  Amp_mm : Inport  OutDataTypeStr=double
  f_Hz : Inport  Port=2
  phi_deg : Inport  Port=3  OutDataTypeStr=double
  Add : Sum
  Clock : Clock
  Constant : Constant  Value=2
  Constant1 : Constant  Value=3.14159265359
  Constant2 : Constant  Value=3.14159265359
  Constant3 : Constant  Value=180
  Constant4 : Constant  Value=1e-3
  Math Reciprocal : Math  Operator=reciprocal  SignedPower=on
  Product : Product  Inputs=4
  Product{1..4} (4 alike) : Product
  Sin : Trigonometry
  r : Outport
  wires:
  Constant1/1 -> Product/2
  Constant/1 -> Product/1
  f_Hz/1 -> Product/3
  phi_deg/1 -> Product1/1
  Constant2/1 -> Product2/1
  Constant3/1 -> Math Reciprocal/1
  Math Reciprocal/1 -> Product2/2
  Product2/1 -> Product1/2
  Clock/1 -> Product/4
  Product/1 -> Sin/1
  Sin/1 -> Product3/2
  Product1/1 -> Add/2
  Product3/1 -> Add/1
  Add/1 -> r/1
  Amp_mm/1 -> Product4/2
  Product4/1 -> Product3/1
  Constant4/1 -> Product4/1

== system phdMain/Subsystem1/Fault_Injection ==
  Constant : Constant  Value=0
  fs : Outport  OutDataTypeStr=double
  wires:
  Constant/1 -> fs/1

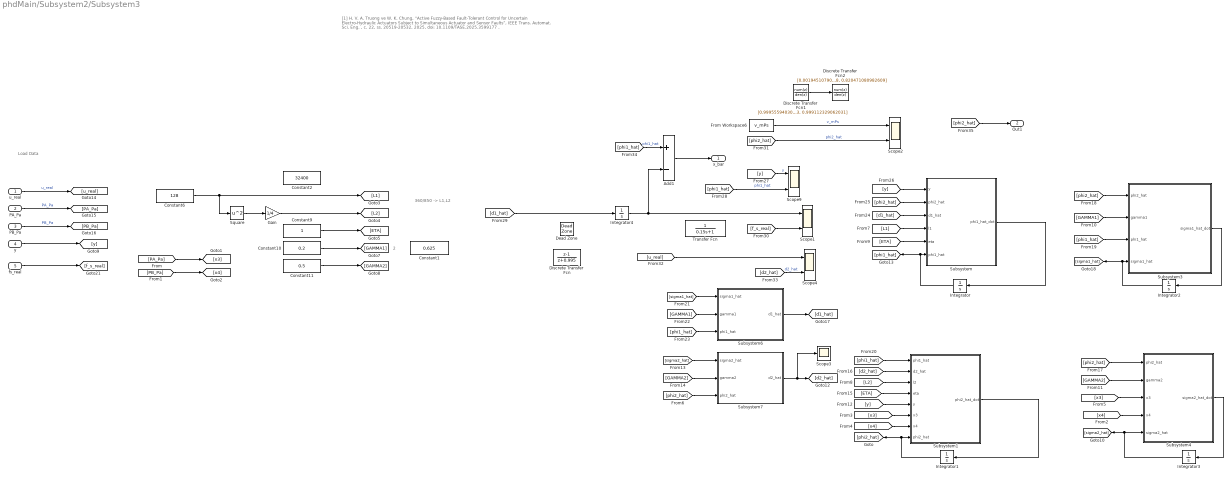
== system phdMain/Subsystem2/Subsystem3 ==
  note: [1]
      | H. V. A. Truong ve W. K. Chung, “Active Fuzzy-Based Fault-Tolerant Control for Uncertain Electro-Hydraulic Actuators Subject to Simultaneous Actuator and Sensor Faults”, IEEE Trans. Automat. Sci. Eng. , c. 22, ss. 20519-20532, 2025, doi: 10.1109/TASE.2025.3599177 .
  note: 2
  note: 360/850 -> L1,L2
  note: Load Data
  u_real : Inport
  PA_Pa : Inport  Port=2
  PB_Pa : Inport  Port=3
  y : Inport  Port=4
  fs_real : Inport  Port=5
  Add1 : Sum  Inputs=+-
  Constant1 : Constant  Value=0.625
  Constant10 : Constant  Value=0.2
  Constant11 : Constant  Value=0.5
  Constant2 : Constant  Value=32400
  Constant6 : Constant  Value=128
  Constant9 : Constant
  Dead Zone : DeadZone  LowerValue=-0.01  UpperValue=0.01
  Discrete Transfer Fcn : DiscreteTransferFcn  Numerator=[1 -1]  Denominator=[1 0.995]
  Discrete Transfer Fcn1 : DiscreteTransferFcn  Numerator=[0.999555940307616, -1.999111880615232, 0.999555940307616]  Denominator=[1.000000000000000, -1.999111432168433, 0.999112329062031]
  Discrete Transfer Fcn2 : DiscreteTransferFcn  Numerator=[0.001945107908955, 0.003890215817911, 0.001945107908955]  Denominator=[1.000000000000000, -1.812690649346788, 0.820471080982609]
  From Workspace6 : FromWorkspace  VariableName=v_mPs
  Gain : Gain  Gain=1/4
  Integrator{,1..4} (5 alike) : Integrator
  Scope{1..2,4,9} (4 alike) : Scope  NumInputPorts=2
  Scope3 : Scope
  Square : Math  Operator=square
  Subsystem : Subsystem
  Subsystem1 : Subsystem
  Subsystem3 : Subsystem
  Subsystem4 : Subsystem
  Subsystem6 : Subsystem
  Subsystem7 : Subsystem
  Transfer Fcn : TransferFcn  Denominator=[0.15 1]
  x_bar : Outport
  Out1 : Outport  Port=2
  wires:
  [u_real] -> Scope4/1
  Subsystem4/1(sigma2_hat_dot) -> Integrator3/1
  Constant6/1 -> Square/1, [L1]
  [y] -> Subsystem/1(y)
  Constant9/1 -> [ETA]
  [GAMMA2] -> Subsystem7/2(gamma2)
  [GAMMA1] -> Subsystem3/2(gamma1)
  Subsystem/1(phi1_hat_dot) -> Integrator/1
  Gain/1 -> [L2]
  [GAMMA1] -> Subsystem6/2(gamma1)
  [y] -> Subsystem1/5(y)
  Constant10/1 -> [GAMMA1]
  y/1 -> [y]
  [GAMMA2] -> Subsystem4/2(gamma2)
  Subsystem7/1(d2_hat) -> Scope3/1, [d2_hat]
  [L2] -> Subsystem1/3(l2)
  Subsystem6/1(d1_hat) -> [d1_hat]
  [phi1_hat] -> Subsystem3/3(phi1_hat)
  [ETA] -> Subsystem/5(eta)
  [phi1_hat] -> Scope9/2  "phi1_hat"
  Integrator/1 -> [phi1_hat], Subsystem/6(phi1_hat)
  [d2_hat] -> Subsystem1/2(d2_hat)
  Constant11/1 -> [GAMMA2]
  [d2_hat] -> Scope4/2  "d2_hat"
  [phi2_hat] -> Subsystem7/3(phi2_hat)
  [y] -> Scope9/1  "y"
  [phi2_hat] -> Subsystem4/1(phi2_hat)
  [sigma1_hat] -> Subsystem6/1(sigma1_hat)
  [L1] -> Subsystem/4(l1)
  Integrator2/1 -> [sigma1_hat], Subsystem3/4(sigma1_hat)
  [PA_Pa] -> [x3]
  [x3] -> Subsystem1/6(x3)
  PB_Pa/1 -> [PB_Pa]  "PB_Pa"
  u_real/1 -> [u_real]  "u_real"
  Subsystem3/1(sigma1_hat_dot) -> Integrator2/1
  [ETA] -> Subsystem1/4(eta)
  [phi1_hat] -> Subsystem6/3(phi1_hat)
  Integrator3/1 -> Subsystem4/5(sigma2_hat), [sigma2_hat]
  [sigma2_hat] -> Subsystem7/1(sigma2_hat)
  [x3] -> Subsystem4/3(x3)
  [x4] -> Subsystem4/4(x4)
  [d1_hat] -> Subsystem/3(d1_hat)
  From Workspace6/1 -> Scope2/1  "v_mPs"
  [phi1_hat] -> Subsystem1/1(phi1_hat)
  [phi2_hat] -> Subsystem/2(phi2_hat)
  [phi2_hat] -> Subsystem3/1(phi2_hat)
  [x4] -> Subsystem1/7(x4)
  PA_Pa/1 -> [PA_Pa]  "PA_Pa"
  [PB_Pa] -> [x4]
  [phi1_hat] -> Add1/1  "phi1_hat"
  Add1/1 -> x_bar/1
  fs_real/1 -> [f_s_real]
  [phi2_hat] -> Out1/1
  Subsystem1/1(phi2_hat_dot) -> Integrator1/1
  Integrator1/1 -> Subsystem1/8(phi2_hat), [phi2_hat]
  Square/1 -> Gain/1
  [d1_hat] -> Integrator4/1
  Integrator4/1 -> Scope1/1, Add1/2
  [f_s_real] -> Scope1/2
  Discrete Transfer Fcn1/1 -> Discrete Transfer Fcn2/1
  [phi2_hat] -> Scope2/2  "phi2_hat"

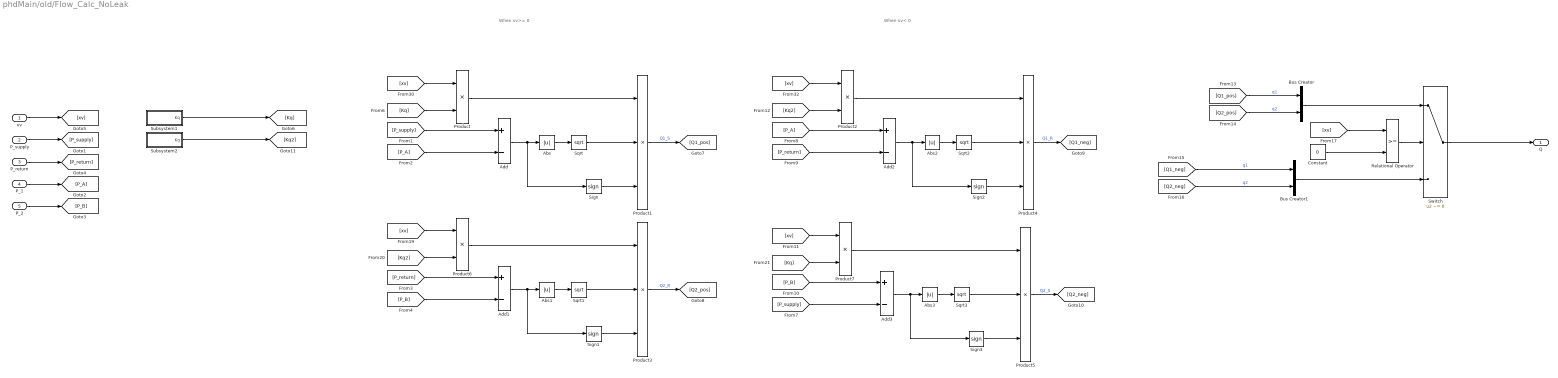
== system phdMain/old/Flow_Calc_NoLeak ==
  note: When xv< 0
  note: When xv>= 0
  xv : Inport  OutDataTypeStr=double
  P_supply : Inport  Port=2  OutDataTypeStr=double
  P_return : Inport  Port=3  OutDataTypeStr=double
  P_1 : Inport  Port=4  OutDataTypeStr=double
  P_2 : Inport  Port=5  OutDataTypeStr=double
  Abs{,1..3} (4 alike) : Abs  SaturateOnIntegerOverflow=off
  Add{,1..3} (4 alike) : Sum  Inputs=+-
  Bus Creator : BusCreator  Inputs=2
  Bus Creator1 : BusCreator  Inputs=2
  Constant : Constant  Value=0  OutDataTypeStr=double
  Product{,2,6..7} (4 alike) : Product
  Product{1,3..5} (4 alike) : Product  Inputs=3
  Relational Operator : RelationalOperator  OutDataTypeStr=boolean  RndMeth=Simplest  InputSameDT=off
  Sign{,1..3} (4 alike) : Signum
  Sqrt{,1..3} (4 alike) : Sqrt
  Subsystem1 : Subsystem
  Subsystem2 : Subsystem
  Switch : Switch  Criteria=u2 ~= 0  SaturateOnIntegerOverflow=off  InputSameDT=off
  Q : Outport  OutDataTypeStr=double
  wires:
  Subsystem2/1(Kq) -> [Kq2]
  Subsystem1/1(Kq) -> [Kq]
  Product5/1 -> [Q2_neg]  "Q2_S"
  Product4/1 -> [Q1_neg]  "Q1_R"
  Product3/1 -> [Q2_pos]  "Q2_R"
  Product1/1 -> [Q1_pos]  "Q1_S"
  Switch/1 -> Q/1
  [xv] -> Product/1
  [Q1_neg] -> Bus Creator1/1  "q1"
  [Q2_pos] -> Bus Creator/2  "q2"
  Product7/1 -> Product5/1
  [xv] -> Product7/1
  [Kq] -> Product7/2
  Product6/1 -> Product3/1
  [Kq2] -> Product6/2
  [xv] -> Product6/1
  Bus Creator1/1 -> Switch/3
  Bus Creator/1 -> Switch/1
  Relational Operator/1 -> Switch/2
  Constant/1 -> Relational Operator/2
  [xv] -> Relational Operator/1
  [Q2_neg] -> Bus Creator1/2  "q2"
  [Q1_pos] -> Bus Creator/1  "q1"
  [P_supply] -> Add3/2
  [P_B] -> Add3/1
  [P_return] -> Add2/2
  [P_A] -> Add2/1
  Product2/1 -> Product4/1
  Sqrt2/1 -> Product4/2
  Abs2/1 -> Sqrt2/1
  Add2/1 -> Abs2/1, Sign2/1
  Sign2/1 -> Product4/3
  Sign3/1 -> Product5/3
  Add3/1 -> Sign3/1, Abs3/1
  Abs3/1 -> Sqrt3/1
  Sqrt3/1 -> Product5/2
  [Kq2] -> Product2/2
  [xv] -> Product2/1
  xv/1 -> [xv]
  P_return/1 -> [P_return]
  P_2/1 -> [P_B]
  P_1/1 -> [P_A]
  P_supply/1 -> [P_supply]
  [P_B] -> Add1/2
  [P_return] -> Add1/1
  [Kq] -> Product/2
  Sqrt1/1 -> Product3/2
  Abs1/1 -> Sqrt1/1
  Add1/1 -> Abs1/1, Sign1/1
  Sign1/1 -> Product3/3
  Sign/1 -> Product1/3
  Add/1 -> Sign/1, Abs/1
  Abs/1 -> Sqrt/1
  Sqrt/1 -> Product1/2
  Product/1 -> Product1/1
  [P_A] -> Add/2
  [P_supply] -> Add/1

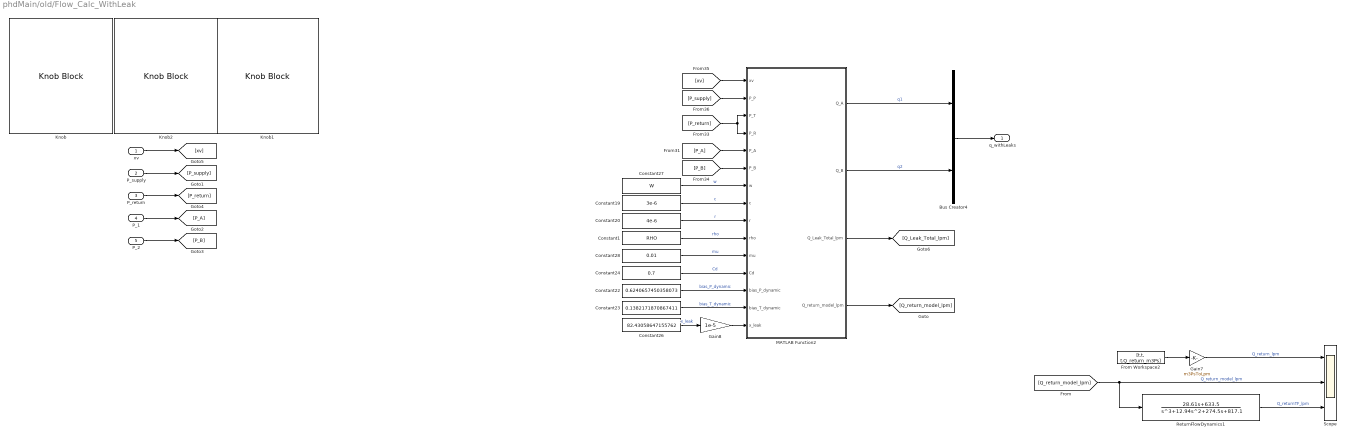
== system phdMain/old/Flow_Calc_WithLeak ==
  xv : Inport  OutDataTypeStr=double
  P_supply : Inport  Port=2  OutDataTypeStr=double
  P_return : Inport  Port=3  OutDataTypeStr=double
  P_1 : Inport  Port=4  OutDataTypeStr=double
  P_2 : Inport  Port=5  OutDataTypeStr=double
  Bus Creator4 : BusCreator  Inputs=2
  Constant1 : Constant  Value=RHO
  Constant19 : Constant  Value=3e-6
  Constant20 : Constant  Value=4e-6
  Constant22 : Constant  Value=0.6240657450358073
  Constant23 : Constant  Value=0.1382171870867411
  Constant24 : Constant  Value=0.7
  Constant26 : Constant  Value=82.43058647155762
  Constant27 : Constant  Value=W
  Constant28 : Constant  Value=0.01
  From Workspace2 : FromWorkspace  VariableName=[t.t, t.Q_return_m3Ps]
  Gain7 : Gain  Gain=m3PsToLpm
  Gain8 : Gain  Gain=1e-5
  Knob : KnobBlock  ScaleMin=0.1  ScaleMax=2
  Knob1 : KnobBlock  ScaleMin=0.1
  Knob2 : KnobBlock  ScaleMin=0.1  ScaleMax=2
  MATLAB Function2 : MATLAB Function  TreatAsAtomicUnit=on
  ReturnFlowDynamics1 : TransferFcn  Numerator=[28.61 633.5]  Denominator=[1 12.94 274.5 817.1]
  Scope : Scope  NumInputPorts=3
  q_withLeaks : Outport  OutDataTypeStr=double
  wires:
  P_supply/1 -> [P_supply]
  P_1/1 -> [P_A]
  P_2/1 -> [P_B]
  P_return/1 -> [P_return]
  xv/1 -> [xv]
  [xv] -> MATLAB Function2/1(xv)
  [P_supply] -> MATLAB Function2/2(P_P)
  [P_return] -> MATLAB Function2/3(P_T), MATLAB Function2/4(P_R)
  [P_A] -> MATLAB Function2/5(P_A)
  [P_B] -> MATLAB Function2/6(P_B)
  Constant27/1 -> MATLAB Function2/7(w)  "w"
  Constant19/1 -> MATLAB Function2/8(c)  "c"
  Constant20/1 -> MATLAB Function2/9(r)  "r"
  Constant1/1 -> MATLAB Function2/10(rho)  "rho"
  Constant28/1 -> MATLAB Function2/11(mu)  "mu"
  Constant24/1 -> MATLAB Function2/12(Cd)  "Cd"
  Constant22/1 -> MATLAB Function2/13(bias_P_dynamic)  "bias_P_dynamic"
  Constant23/1 -> MATLAB Function2/14(bias_T_dynamic)  "bias_T_dynamic"
  From Workspace2/1 -> Gain7/1
  Bus Creator4/1 -> q_withLeaks/1
  MATLAB Function2/1(Q_A) -> Bus Creator4/1  "q1"
  MATLAB Function2/2(Q_B) -> Bus Creator4/2  "q2"
  Constant26/1 -> Gain8/1  "x_leak"
  Gain8/1 -> MATLAB Function2/15(x_leak)
  MATLAB Function2/4(Q_return_model_lpm) -> [Q_return_model_lpm]
  MATLAB Function2/3(Q_Leak_Total_lpm) -> [Q_Leak_Total_lpm]
  Gain7/1 -> Scope/1  "Q_return_lpm"
  ReturnFlowDynamics1/1 -> Scope/3  "Q_returnTF_lpm"
  [Q_return_model_lpm] -> ReturnFlowDynamics1/1, Scope/2  "Q_return_model_lpm"

== system phdMain/old/ServoValve_Dynamics ==
  note: Deadband
  u : Inport  OutDataTypeStr=double
  Convert_SpoolPosition : Subsystem
  Dead Zone : DeadZone  LowerValue=-0.05  UpperValue=0.05
  Subsystem : Subsystem  Commented=on
  Valve Dynamics : TransferFcn  Numerator=[2.0884e+06]  Denominator=[1 2*1*1.4451e+03 2.0884e+06]
  xv : Outport  OutDataTypeStr=double
  wires:
  Dead Zone/1 -> Valve Dynamics/1
  u/1 -> Dead Zone/1
  Convert_SpoolPosition/1(xv) -> xv/1
  Valve Dynamics/1 -> Convert_SpoolPosition/1(u_perc)

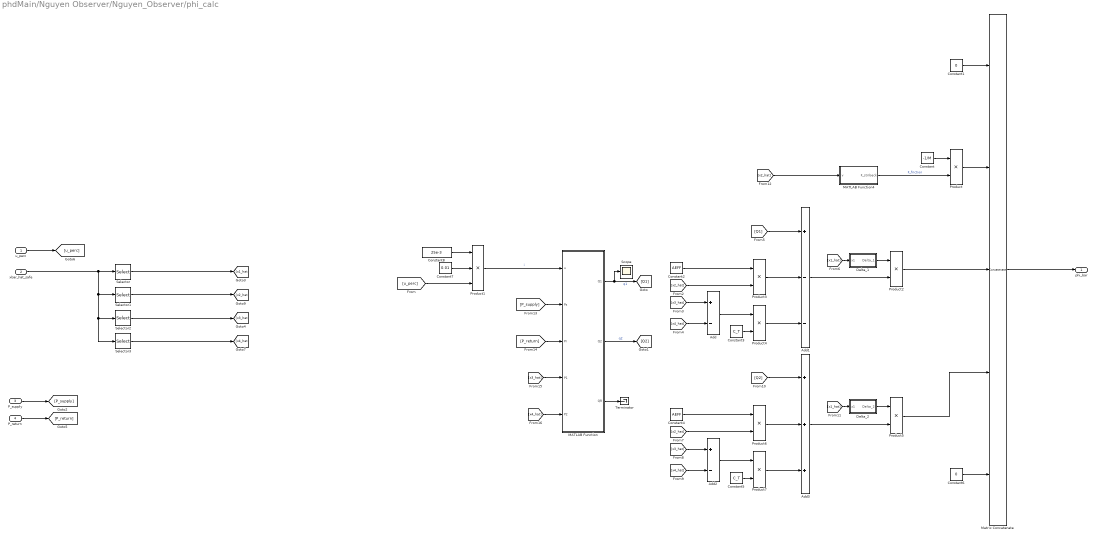
== system phdMain/Nguyen Observer/Nguyen_Observer/phi_calc ==
  u_perc : Inport
  xbar_hat_safe : Inport  Port=2
  P_supply : Inport  Port=3  OutDataTypeStr=double
  P_return : Inport  Port=4  OutDataTypeStr=double
  Add : Sum  Inputs=+-
  Add1 : Sum  Inputs=+--
  Add2 : Sum  Inputs=+-
  Add3 : Sum  Inputs=+++
  Constant : Constant  Value=-1/M
  Constant1 : Constant  Value=0
  Constant2 : Constant  Value=AEFF
  Constant3 : Constant  Value=C_T
  Constant4 : Constant  Value=AEFF
  Constant5 : Constant  Value=C_T
  Constant6 : Constant  Value=0
  Constant7 : Constant  Value=0.01
  Constant8 : Constant  Value=25e-3
  Delta_1 : Subsystem
  Delta_2 : Subsystem
  MATLAB Function : MATLAB Function  TreatAsAtomicUnit=on
  MATLAB Function4 : MATLAB Function  TreatAsAtomicUnit=on
  Matrix Concatenate : Concatenate  NumInputs=5  Mode=Multidimensional array
  Product{,2..7} (7 alike) : Product
  Product1 : Product  Inputs=3
  Scope : Scope
  Selector : Selector  InputPortWidth=5  IndexOptions=Index vector (dialog)  Indices=1  OutputSizes=1
  Selector1 : Selector  InputPortWidth=5  IndexOptions=Index vector (dialog)  Indices=2  OutputSizes=1
  Selector2 : Selector  InputPortWidth=5  IndexOptions=Index vector (dialog)  Indices=3  OutputSizes=1
  Selector3 : Selector  InputPortWidth=5  IndexOptions=Index vector (dialog)  Indices=4  OutputSizes=1
  Terminator : Terminator
  phi_bar : Outport
  wires:
  MATLAB Function4/1(F_stribeck) -> Product/2  "F_friction"
  Constant/1 -> Product/1
  MATLAB Function/1(Q1) -> Scope/1, [Q1]  "q1"
  MATLAB Function/2(Q2) -> [Q2]  "q2"
  [Q1] -> Add1/1
  [x2_hat] -> Product3/2
  [x4_hat] -> Add/2
  [x3_hat] -> Add/1
  Add/1 -> Product4/1
  Constant3/1 -> Product4/2
  Product3/1 -> Add1/2
  Product4/1 -> Add1/3
  Add1/1 -> Product2/2
  Delta_1/1(Delta_1) -> Product2/1
  [x1_hat] -> Delta_1/1(x1)
  [x1_hat] -> Delta_2/1(x1)
  Delta_2/1(Delta_2) -> Product5/1
  Add3/1 -> Product5/2
  Product7/1 -> Add3/3
  Product6/1 -> Add3/2
  Constant5/1 -> Product7/2
  Add2/1 -> Product7/1
  [x3_hat] -> Add2/1
  [x4_hat] -> Add2/2
  [x2_hat] -> Product6/2
  [Q2] -> Add3/1
  Constant6/1 -> Matrix Concatenate/5
  Product5/1 -> Matrix Concatenate/4
  Product/1 -> Matrix Concatenate/2
  Constant1/1 -> Matrix Concatenate/1
  Constant7/1 -> Product1/2
  Constant8/1 -> Product1/1
  Product1/1 -> MATLAB Function/1(u)  "i"
  u_perc/1 -> [u_perc]
  P_return/1 -> [P_return]
  P_supply/1 -> [P_supply]
  [u_perc] -> Product1/3
  [P_supply] -> MATLAB Function/2(Ps)
  [P_return] -> MATLAB Function/3(Pr)
  [x3_hat] -> MATLAB Function/4(P1)
  [x4_hat] -> MATLAB Function/5(P2)
  MATLAB Function/3(QR) -> Terminator/1
  Matrix Concatenate/1 -> phi_bar/1
  Selector/1 -> [x1_hat]
  Selector1/1 -> [x2_hat]
  Selector2/1 -> [x3_hat]
  Selector3/1 -> [x4_hat]
  Constant2/1 -> Product3/1
  Constant4/1 -> Product6/1
  Product2/1 -> Matrix Concatenate/3
  [x2_hat] -> MATLAB Function4/1(v)
  xbar_hat_safe/1 -> Selector3/1, Selector2/1, Selector1/1, Selector/1

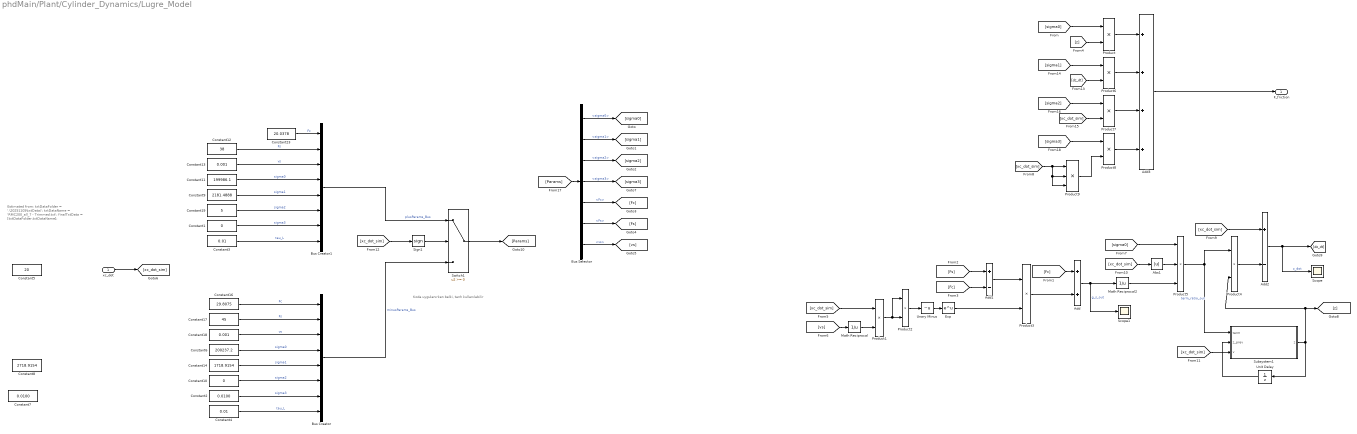
== system phdMain/Plant/Cylinder_Dynamics/Lugre_Model ==
  note: Koda uygulanırken belki, tanh kullanılabilir
  note: Estimated from:
      |
      | txtDataFolder = '.\20251105\txtData\';
      | txtDataName = 'RMC200_all_7 - Trimmed.txt';
      | finalTxtData = [txtDataFolder,txtDataName];
  xc_dot : Inport  OutDataTypeStr=double
  Abs1 : Abs  SaturateOnIntegerOverflow=off
  Add : Sum
  Add1 : Sum  Inputs=+-
  Add2 : Sum  Inputs=+-
  Add3 : Sum  Inputs=++++
  Bus Selector : BusSelector  OutputSignals=sigma0,sigma1,sigma2,sigma3,Fc,Fs,vs
  Bus Creator : BusCreator  Inputs=8
  Bus Creator1 : BusCreator  Inputs=8
  Constant1 : Constant  Value=0  OutDataTypeStr=double
  Constant10 : Constant  Value=0  OutDataTypeStr=double
  Constant11 : Constant  Value=199986.1  OutDataTypeStr=double
  Constant12 : Constant  Value=38  OutDataTypeStr=double
  Constant13 : Constant  Value=0.001  OutDataTypeStr=double
  Constant14 : Constant  Value=1718.9154  OutDataTypeStr=double
  Constant16 : Constant  Value=29.8075  OutDataTypeStr=double
  Constant17 : Constant  Value=45  OutDataTypeStr=double
  Constant18 : Constant  Value=0.001  OutDataTypeStr=double
  Constant19 : Constant  Value=5  OutDataTypeStr=double
  Constant2 : Constant  Value=0.0100  OutDataTypeStr=double
  Constant23 : Constant  Value=20.0378  OutDataTypeStr=double
  Constant3 : Constant  Value=0.01  OutDataTypeStr=double
  Constant4 : Constant  Value=0.01  OutDataTypeStr=double
  Constant5 : Constant  Value=20  OutDataTypeStr=double
  Constant6 : Constant  Value=200237.2  OutDataTypeStr=double
  Constant7 : Constant  Value=0.0100  OutDataTypeStr=double
  Constant8 : Constant  Value=2718.9154  OutDataTypeStr=double
  Constant9 : Constant  Value=2181.4888  OutDataTypeStr=double
  Exp : Math  SignedPower=on
  Math Reciprocal : Math  Operator=reciprocal  SignedPower=on
  Math Reciprocal2 : Math  Operator=reciprocal  SignedPower=on
  Product{,1..4,6..8} (8 alike) : Product
  Product5 : Product  Inputs=3
  Product9 : Product  Inputs=3
  Scope : Scope
  Scope1 : Scope
  Sign1 : Signum
  Subsystem1 : Subsystem
  Switch1 : Switch  SaturateOnIntegerOverflow=off  InputSameDT=off
  Unary Minus : UnaryMinus
  Unit Delay : UnitDelay  SampleTime=-1  HasFrameUpgradeWarning=on
  F_friction : Outport
  wires:
  Constant18/1 -> Bus Creator/3  "vs"
  Constant13/1 -> Bus Creator1/3  "vs"
  Constant12/1 -> Bus Creator1/2  "Fs"
  Constant17/1 -> Bus Creator/2  "Fs"
  Constant14/1 -> Bus Creator/5  "sigma1"
  Constant6/1 -> Bus Creator/4  "sigma0"
  Constant10/1 -> Bus Creator/6  "sigma2"
  Constant16/1 -> Bus Creator/1  "Fc"
  Constant9/1 -> Bus Creator1/5  "sigma1"
  Constant11/1 -> Bus Creator1/4  "sigma0"
  Constant19/1 -> Bus Creator1/6  "sigma2"
  Product7/1 -> Add3/3
  Product6/1 -> Add3/2
  [sigma2] -> Product7/1
  [xc_dot_sim] -> Product7/2
  [dz_dt] -> Product6/2
  [sigma1] -> Product6/1
  Product/1 -> Add3/1
  [z] -> Product/2
  [sigma0] -> Product5/1
  Abs1/1 -> Product5/2
  Add/1 -> Math Reciprocal2/1, Scope1/1  "g_s_out"
  [xc_dot_sim] -> Abs1/1
  Add1/1 -> Product3/1
  Unary Minus/1 -> Exp/1
  Product2/1 -> Unary Minus/1
  Product1/1 -> Product2/2, Product2/1
  [xc_dot_sim] -> Product1/1
  Math Reciprocal/1 -> Product1/2
  [vs] -> Math Reciprocal/1
  [Fc] -> Add1/2
  [Fs] -> Add1/1
  [Fc] -> Add/1
  [sigma0] -> Product/1
  Product3/1 -> Add/2
  [xc_dot_sim] -> Sign1/1
  Bus Creator1/1 -> Switch1/1  "plusParams_Bus"
  Bus Creator/1 -> Switch1/3  "minusParams_Bus"
  Switch1/1 -> [Params]
  [Params] -> Bus Selector/1
  Bus Selector/1 -> [sigma0]  "<sigma0>"
  Bus Selector/2 -> [sigma1]  "<sigma1>"
  Bus Selector/3 -> [sigma2]  "<sigma2>"
  Bus Selector/5 -> [Fc]  "<Fc>"
  Bus Selector/6 -> [Fs]  "<Fs>"
  Bus Selector/7 -> [vs]  "<vs>"
  Math Reciprocal2/1 -> Product5/3
  Exp/1 -> Product3/2
  Add2/1 -> Scope/1, [dz_dt]  "z_dot"
  Sign1/1 -> Switch1/2
  [xc_dot_sim] -> Add2/1
  Subsystem1/1(z) -> Product4/2, [z], Unit Delay/1
  [xc_dot_sim] -> Subsystem1/3(v)
  Unit Delay/1 -> Subsystem1/2(z_prev)
  Product5/1 -> Subsystem1/1(term), Product4/1  "term_ratio_out"
  Product4/1 -> Add2/2
  Add3/1 -> F_friction/1
  Constant1/1 -> Bus Creator1/7  "sigma3"
  Constant2/1 -> Bus Creator/7  "sigma3"
  Constant3/1 -> Bus Creator1/8  "tau_L"
  Constant4/1 -> Bus Creator/8  "tau_L"
  [sigma3] -> Product8/1
  Product8/1 -> Add3/4
  [xc_dot_sim] -> Product9/2, Product9/3, Product9/1
  Product9/1 -> Product8/2
  Bus Selector/4 -> [sigma3]  "<sigma3>"
  xc_dot/1 -> [xc_dot_sim]
  Constant23/1 -> Bus Creator1/1  "Fc"
